simulink model "pidemp"  (Simulink 3.00)
settings: Solver=ode45  SolverMode=SingleTasking  StartTime=0.0  StopTime=100  MaxStep=.010  RelTol=1e-3  AbsTol=1e-3
undefined symbols (not defined in the file or in its folder): at, bt, ct, dt
settings Model: TimeSaveName=t  SaveOutput=off

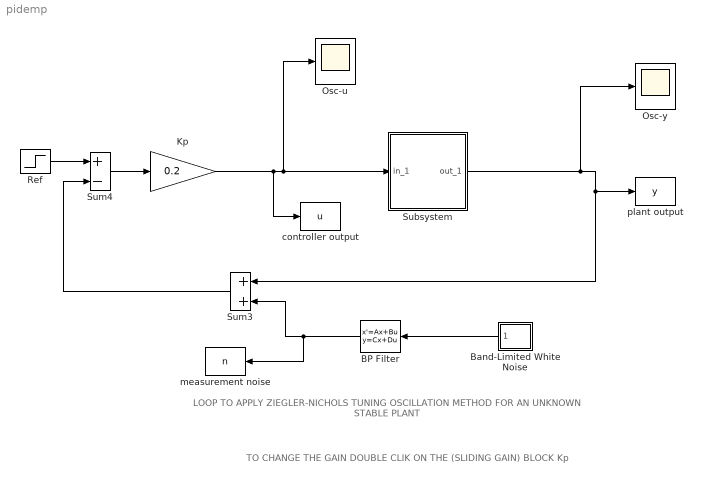
== system pidemp ==
  note: LOOP TO APPLY ZIEGLER-NICHOLS TUNING OSCILLATION METHOD
      | FOR AN UNKNOWN STABLE PLANT
  note: TO CHANGE THE GAIN DOUBLE CLIK ON THE (SLIDING GAIN) BLOCK Kp
  "BP Filter " : StateSpace  Orientation=left  A=at  B=bt  C=ct  D=dt  X0=0  mask(buttap,lp2bp){@1=2, @2=2, @3=4}
      mask prompts: @1 "Center frequency (rad/sec)"; @2 "Bandwidth (rad/sec):"; @3 "Order"
      mask help:
      | Analog Butterworth band pass filter.
      |
      | (Requires Signal Processing Toolbox)
      mask init:
      | [at,bt,ct,dt,w,mag]=filtm('buttap','lp2bp',@1,@2,50,@3);
      mask Help: Butterworth band pass filter using MATLAB's butter and lp2bp command.
      mask Display: plot(w,mag)
  Band-Limited White Noise : Subsystem  Orientation=left  mask(Continuous White Noise.){@1=[0.1], @2=0.1, @3=[23341]}
      mask prompts: @1 "Noise Power:"; @2 "Sample Time:"; @3 "Seed"
      mask help:
      | White noise for continuous (s-domain) systems.
      | Band-limited using zero-order-hold.
      mask init:
      | Cov = @1; Ts = @2; seed = @3; r = rand(1,12); r2 = [r(1),r;r,r(12)]; t =[1:13;1:13];
      mask Help: Implemented using white noise into Zero-Order Hold block. The seed and power can be vectors of the same length to produce a vector of white noise sources. For faster simulation, set sample time to the highest value possible but in accordance with the fastest dynamics of system.
      mask Display: plot(t(:),r2(:))
  Kp : Gain  LoadFcn=slideg Load  Gain=0.2  SaturateOnIntegerOverflow=on  mask{@1=0, @2=0.2, @3=5}
      mask prompts: @1 "Low"; @2 "Gain"; @3 "High"
      settings: CopyFcn=slideg Copy  DeleteFcn=slideg DeleteBlock  NameChangeFcn=slideg NameChange  OpenFcn=slideg Open  ParentCloseFcn=slideg ParentClose
      mask Display: disp('0.2')
  Osc-u : Scope
      settings: TickLabels=on  TimeRange=100.000000  YMin=-2.000000  YMax=2.000000  SaveToWorkspace=off  SaveName=ScopeData  DataFormat=Matrix
  Osc-y : Scope
      settings: TickLabels=on  TimeRange=100.000000  YMin=-2  YMax=2  SaveToWorkspace=off  SaveName=ScopeData  DataFormat=Matrix
  Ref : Step  Time=10  Before=0  After=2  SampleTime=0
  Subsystem : Subsystem  mask(buttap){lows=-10, upps=10, bw=1, ord=3}
      mask prompts: lows "Lower limit saturation value"; upps "Upper limit saturation value"; bw "Cutoff frequency (rad/sec)"; ord "Order"
      mask help:
      | Analog Butterworth low pass filter.
      |
      | (Requires Signal Processing Toolbox)
      mask init:
      | [z,p,k]=buttap(ord); z=bw*z; p=bw*p; k=real(prod(-p)); [num,den]=zp2tf(z,p,k); w=logspace(log10(bw/10),log10(10*bw),20); h=freqs(num,den,w);
      mask Help: Butterworth low pass filter using MATLAB's butter command.
      mask Display: plot(20*log10(w),20*log10(abs(h)))
  Sum3 : Sum  Orientation=left  Inputs=++  SaturateOnIntegerOverflow=on
  Sum4 : Sum  Inputs=+-  SaturateOnIntegerOverflow=on
  controller output : ToWorkspace  VariableName=u  SampleTime=0  SaveFormat=Matrix
      settings: Buffer=10000
  measurement noise : ToWorkspace  VariableName=n  SampleTime=0  SaveFormat=Matrix
      settings: Buffer=10000
  plant output : ToWorkspace  VariableName=y  SampleTime=0  SaveFormat=Matrix
      settings: Buffer=10000
  wires:
  Sum4/1 -> Kp/1
  Ref/1 -> Sum4/1
  Band-Limited White Noise/1(Out_1) -> "BP Filter "/1
  Subsystem/1(out_1) -> Osc-y/1, Sum3/1, plant output/1
  "BP Filter "/1 -> Sum3/2, measurement noise/1
  Kp/1 -> Subsystem/1(in_1), Osc-u/1, controller output/1
  Sum3/1 -> Sum4/2

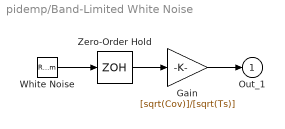
== system pidemp/Band-Limited White Noise ==
  Gain : Gain  Gain=[sqrt(Cov)]/[sqrt(Ts)]  SaturateOnIntegerOverflow=on
  White Noise : RandomNumber  Mean=0  Variance=1  Seed=seed  SampleTime=0
  Zero-Order Hold : ZeroOrderHold  SampleTime=Ts
  Out_1 : Outport  Port=1  InitialOutput=0
  wires:
  White Noise/1 -> Zero-Order Hold/1
  Gain/1 -> Out_1/1
  Zero-Order Hold/1 -> Gain/1

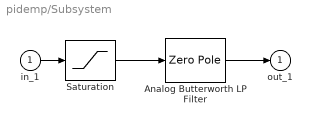
== system pidemp/Subsystem ==
  in_1 : Inport  Port=1  PortWidth=-1  SampleTime=-1  DataType=auto
      settings: SignalType=auto
  Analog Butterworth LP Filter : ZeroPole  Zeros=z  Poles=p  Gain=k
  Saturation : Saturate  UpperLimit=upps  LowerLimit=lows
  out_1 : Outport  Port=1  InitialOutput=0
  wires:
  Saturation/1 -> Analog Butterworth LP Filter/1
  in_1/1 -> Saturation/1
  Analog Butterworth LP Filter/1 -> out_1/1
